simulink model "sm_aileron_actuator_2"  (R2022b)
settings: Solver=FixedStepAuto  StartTime=0.0  StopTime=50.0  FixedStep=0.01  RelTol=1e-3  AbsTol=1e-4  EnableMultiTasking=on
PostLoadFcn:
  | warning('off','sm:sli:setup:compile:LocalSolverNotSupported')
StartFcn:
  | tic
StopFcn:
  | Elapsed_Sim_Time = toc;
model workspace: external: MATLAB File aileronAssembly_DataFile.m (data not in the file)
undefined symbols (not defined in the file or in its folder): AAC_Param, ang2Ext_coeff, Ki, Ki_scaling_elec, Kp, Leadscrew, motor_friction, R7_sctrl, sigbuilder_block, sm_aileron_actuator_lib, smiData, X, Y, Z
libraries: sm_lib x608, fl_lib x380, ee_lib x103, nesl_utility x87, sh_lib x7, sdl_lib x3, simulink x2, slpidlib x2
(part 22 of 22)

== system sm_aileron_actuator_2/Actuator/Electric/Leadscrew 2/Control/Circuit/Current Controller/PS2V ==
  Controlled Voltage Source : fl_lib/Electrical/Electrical Sources/Controlled Voltage Source
  Electrical Reference : fl_lib/Electrical/Electrical Elements/Electrical Reference
  PS : PMIOPort  Side=Right
  V : PMIOPort  Port=2  Side=Left
  connections:
  V/RConn1 -- Controlled Voltage Source/LConn1
  PS/RConn1 -- Controlled Voltage Source/RConn1
  Electrical Reference/LConn1 -- Controlled Voltage Source/RConn2

== system sm_aileron_actuator_2/Actuator/Electric/Leadscrew 2/Control/Simulink/Current Controller/SL2V_1 ==
  SL : Inport
  Controlled Voltage Source : fl_lib/Electrical/Electrical Sources/Controlled Voltage Source
  Electrical Reference : fl_lib/Electrical/Electrical Elements/Electrical Reference
  Simulink-PS Converter : nesl_utility/Simulink-PS Converter  PhysicalDomain=network_engine_domain  SubClassName=ps_input  LeftPortType=input  RightPortType=output  PseudoPeriodic=off  Frequencies=[]  NoiseDistribution=none  NoiseParameters=[]  Unit=V  AffineConversion=off  FilteringAndDerivatives=zero  SimscapeFilterOrder=1  InputFilterTimeConstant=0.005  UdotUserProvided=0
  V : PMIOPort  Side=Right
  wires:
  SL/1 -> Simulink-PS Converter/1
  connections:
  Simulink-PS Converter/RConn1 -- Controlled Voltage Source/RConn1
  V/RConn1 -- Controlled Voltage Source/LConn1
  Electrical Reference/LConn1 -- Controlled Voltage Source/RConn2

== system sm_aileron_actuator_2/Actuator/Electric/Leadscrew 2/Control/Simulink/Current Controller/SL2V_2 ==
  SL : Inport
  Controlled Voltage Source : fl_lib/Electrical/Electrical Sources/Controlled Voltage Source
  Electrical Reference : fl_lib/Electrical/Electrical Elements/Electrical Reference
  Simulink-PS Converter : nesl_utility/Simulink-PS Converter  PhysicalDomain=network_engine_domain  SubClassName=ps_input  LeftPortType=input  RightPortType=output  PseudoPeriodic=off  Frequencies=[]  NoiseDistribution=none  NoiseParameters=[]  Unit=V  AffineConversion=off  FilteringAndDerivatives=zero  SimscapeFilterOrder=1  InputFilterTimeConstant=0.005  UdotUserProvided=0
  V : PMIOPort  Side=Right
  wires:
  SL/1 -> Simulink-PS Converter/1
  connections:
  Electrical Reference/LConn1 -- Controlled Voltage Source/RConn2
  V/RConn1 -- Controlled Voltage Source/LConn1
  Simulink-PS Converter/RConn1 -- Controlled Voltage Source/RConn1

== system sm_aileron_actuator_2/Actuator/Electric/Leadscrew 2/Hall Effect Sensor/Detailed Sensor/PIC Decoder/Pulse decode ==
  A : Inport
  B : Inport  Port=2
  Clock : Clock
  Constant : Constant  Value=0.5
  Sign : Signum
  Sum1 : Sum  Inputs=|-+
  Triggered Subsystem : Subsystem  TreatAsAtomicUnit=on
  Pulse frequency : Outport  VectorParamsAs1DForOutWhenUnconnected=off
  Direction : Outport  Port=2  VectorParamsAs1DForOutWhenUnconnected=off
  Pulse count : Outport  Port=3  VectorParamsAs1DForOutWhenUnconnected=off
  wires:
  Constant/1 -> Sum1/2
  Sum1/1 -> Sign/1
  B/1 -> Sum1/1
  Sign/1 -> Triggered Subsystem/1(sign)
  A/1 -> Triggered Subsystem/Trigger
  Triggered Subsystem/1(Pulse count) -> Pulse count/1
  Clock/1 -> Triggered Subsystem/2(clk)
  Triggered Subsystem/2(Pulse frequency) -> Pulse frequency/1
  Triggered Subsystem/3(Direction) -> Direction/1

== system sm_aileron_actuator_2/Actuator/Electric/Leadscrew 2/Hall Effect Sensor/Detailed Sensor/PIC Decoder/V2SL_1 ==
  Electrical Reference1 : fl_lib/Electrical/Electrical Elements/Electrical Reference
  PS-Simulink Converter 2 : nesl_utility/PS-Simulink Converter  PhysicalDomain=network_engine_domain  SubClassName=ps_output  LeftPortType=input  RightPortType=output  PseudoPeriodic=off  Frequencies=[]  VectorFormat=1-D array  Unit=V  AffineConversion=off
  V2logic : Gain  Gain=0.2
  Voltage Sensor : fl_lib/Electrical/Electrical Sensors/Voltage Sensor
  V : PMIOPort  Side=Left
  SL : Outport  VectorParamsAs1DForOutWhenUnconnected=off
  wires:
  V2logic/1 -> SL/1
  PS-Simulink Converter 2/1 -> V2logic/1
  connections:
  Voltage Sensor/RConn1 -- PS-Simulink Converter 2/LConn1
  V/RConn1 -- Voltage Sensor/LConn1
  Voltage Sensor/RConn2 -- Electrical Reference1/LConn1

== system sm_aileron_actuator_2/Actuator/Electric/Leadscrew 2/Hall Effect Sensor/Detailed Sensor/PIC Decoder/V2SL_2 ==
  Electrical Reference1 : fl_lib/Electrical/Electrical Elements/Electrical Reference
  PS-Simulink Converter 2 : nesl_utility/PS-Simulink Converter  PhysicalDomain=network_engine_domain  SubClassName=ps_output  LeftPortType=input  RightPortType=output  PseudoPeriodic=off  Frequencies=[]  VectorFormat=1-D array  Unit=V  AffineConversion=off
  V2logic : Gain  Gain=0.2
  Voltage Sensor : fl_lib/Electrical/Electrical Sensors/Voltage Sensor
  V : PMIOPort  Side=Left
  SL : Outport  VectorParamsAs1DForOutWhenUnconnected=off
  wires:
  PS-Simulink Converter 2/1 -> V2logic/1
  V2logic/1 -> SL/1
  connections:
  Voltage Sensor/RConn2 -- Electrical Reference1/LConn1
  V/RConn1 -- Voltage Sensor/LConn1
  Voltage Sensor/RConn1 -- PS-Simulink Converter 2/LConn1

== system sm_aileron_actuator_2/Actuator/Electric/Leadscrew 2/Motor Driver/Circuit/LegNl/Sensor Voltage ==
  Goto : Goto  Commented=on  GotoTag=Vds_M2  TagVisibility=global
  PS-Simulink : nesl_utility/PS-Simulink Converter  PhysicalDomain=network_engine_domain  SubClassName=ps_output  LeftPortType=input  RightPortType=output  PseudoPeriodic=off  Frequencies=[]  VectorFormat=1-D array  Unit=V  AffineConversion=off
  Voltage Sensor : fl_lib/Electrical/Electrical Sensors/Voltage Sensor
  + : PMIOPort  Side=Left
  - : PMIOPort  Port=2  Side=Right
  wires:
  PS-Simulink/1 -> Goto/1
  connections:
  -/RConn1 -- Voltage Sensor/RConn2
  +/RConn1 -- Voltage Sensor/LConn1
  Voltage Sensor/RConn1 -- PS-Simulink/LConn1

== system sm_aileron_actuator_2/Actuator/Electric/Leadscrew 2/Motor Driver/Circuit/LegNu/Sensor Voltage ==
  Goto : Goto  Commented=on  GotoTag=Vds_M4  TagVisibility=global
  PS-Simulink : nesl_utility/PS-Simulink Converter  PhysicalDomain=network_engine_domain  SubClassName=ps_output  LeftPortType=input  RightPortType=output  PseudoPeriodic=off  Frequencies=[]  VectorFormat=1-D array  Unit=V  AffineConversion=off
  Voltage Sensor : fl_lib/Electrical/Electrical Sensors/Voltage Sensor
  + : PMIOPort  Side=Left
  - : PMIOPort  Port=2  Side=Right
  wires:
  PS-Simulink/1 -> Goto/1
  connections:
  Voltage Sensor/RConn1 -- PS-Simulink/LConn1
  +/RConn1 -- Voltage Sensor/LConn1
  -/RConn1 -- Voltage Sensor/RConn2

== system sm_aileron_actuator_2/Actuator/Electric/Leadscrew 2/Motor Driver/Circuit/LegPl/Sensor Voltage ==
  Goto : Goto  Commented=on  GotoTag=Vds_M1  TagVisibility=global
  PS-Simulink : nesl_utility/PS-Simulink Converter  PhysicalDomain=network_engine_domain  SubClassName=ps_output  LeftPortType=input  RightPortType=output  PseudoPeriodic=off  Frequencies=[]  VectorFormat=1-D array  Unit=V  AffineConversion=off
  Voltage Sensor : fl_lib/Electrical/Electrical Sensors/Voltage Sensor
  + : PMIOPort  Side=Left
  - : PMIOPort  Port=2  Side=Right
  wires:
  PS-Simulink/1 -> Goto/1
  connections:
  Voltage Sensor/RConn1 -- PS-Simulink/LConn1
  +/RConn1 -- Voltage Sensor/LConn1
  -/RConn1 -- Voltage Sensor/RConn2

== system sm_aileron_actuator_2/Actuator/Electric/Leadscrew 2/Motor Driver/Circuit/LegPu/Sensor Pwr ==
  Goto1 : Goto  Commented=on  GotoTag=Power_M3  TagVisibility=global
  PS-Simulink : nesl_utility/PS-Simulink Converter  PhysicalDomain=network_engine_domain  SubClassName=ps_output  LeftPortType=input  RightPortType=output  PseudoPeriodic=off  Frequencies=[]  VectorFormat=1-D array  Unit=W  AffineConversion=off
  Power Sensor : ee_lib/Sensors & Transducers/Power Sensor  measurement_type=1  averaging_period=1e-4 s
  S : PMIOPort  Side=Right
  + : PMIOPort  Port=2  Side=Left
  - : PMIOPort  Port=3  Side=Left
  wires:
  PS-Simulink/1 -> Goto1/1
  connections:
  PS-Simulink/LConn1 -- Power Sensor/RConn1
  Power Sensor/LConn1 -- S/RConn1
  Power Sensor/LConn3 -- -/RConn1
  Power Sensor/LConn2 -- +/RConn1

== system sm_aileron_actuator_2/Actuator/Electric/Leadscrew 2/Motor Driver/Circuit/LegPu/Sensor Voltage ==
  Goto : Goto  Commented=on  GotoTag=Vds_M3  TagVisibility=global
  PS-Simulink : nesl_utility/PS-Simulink Converter  PhysicalDomain=network_engine_domain  SubClassName=ps_output  LeftPortType=input  RightPortType=output  PseudoPeriodic=off  Frequencies=[]  VectorFormat=1-D array  Unit=V  AffineConversion=off
  Voltage Sensor : fl_lib/Electrical/Electrical Sensors/Voltage Sensor
  + : PMIOPort  Side=Left
  - : PMIOPort  Port=2  Side=Right
  wires:
  PS-Simulink/1 -> Goto/1
  connections:
  -/RConn1 -- Voltage Sensor/RConn2
  +/RConn1 -- Voltage Sensor/LConn1
  Voltage Sensor/RConn1 -- PS-Simulink/LConn1

== system sm_aileron_actuator_2/Actuator/Electric/Leadscrew 3/Control/Circuit/Current Controller/PS2V ==
  Controlled Voltage Source : fl_lib/Electrical/Electrical Sources/Controlled Voltage Source
  Electrical Reference : fl_lib/Electrical/Electrical Elements/Electrical Reference
  PS : PMIOPort  Side=Right
  V : PMIOPort  Port=2  Side=Left
  connections:
  V/RConn1 -- Controlled Voltage Source/LConn1
  PS/RConn1 -- Controlled Voltage Source/RConn1
  Electrical Reference/LConn1 -- Controlled Voltage Source/RConn2

== system sm_aileron_actuator_2/Actuator/Electric/Leadscrew 3/Control/Simulink/Current Controller/SL2V_1 ==
  SL : Inport
  Controlled Voltage Source : fl_lib/Electrical/Electrical Sources/Controlled Voltage Source
  Electrical Reference : fl_lib/Electrical/Electrical Elements/Electrical Reference
  Simulink-PS Converter : nesl_utility/Simulink-PS Converter  PhysicalDomain=network_engine_domain  SubClassName=ps_input  LeftPortType=input  RightPortType=output  PseudoPeriodic=off  Frequencies=[]  NoiseDistribution=none  NoiseParameters=[]  Unit=V  AffineConversion=off  FilteringAndDerivatives=zero  SimscapeFilterOrder=1  InputFilterTimeConstant=0.005  UdotUserProvided=0
  V : PMIOPort  Side=Right
  wires:
  SL/1 -> Simulink-PS Converter/1
  connections:
  Simulink-PS Converter/RConn1 -- Controlled Voltage Source/RConn1
  V/RConn1 -- Controlled Voltage Source/LConn1
  Electrical Reference/LConn1 -- Controlled Voltage Source/RConn2

== system sm_aileron_actuator_2/Actuator/Electric/Leadscrew 3/Control/Simulink/Current Controller/SL2V_2 ==
  SL : Inport
  Controlled Voltage Source : fl_lib/Electrical/Electrical Sources/Controlled Voltage Source
  Electrical Reference : fl_lib/Electrical/Electrical Elements/Electrical Reference
  Simulink-PS Converter : nesl_utility/Simulink-PS Converter  PhysicalDomain=network_engine_domain  SubClassName=ps_input  LeftPortType=input  RightPortType=output  PseudoPeriodic=off  Frequencies=[]  NoiseDistribution=none  NoiseParameters=[]  Unit=V  AffineConversion=off  FilteringAndDerivatives=zero  SimscapeFilterOrder=1  InputFilterTimeConstant=0.005  UdotUserProvided=0
  V : PMIOPort  Side=Right
  wires:
  SL/1 -> Simulink-PS Converter/1
  connections:
  Electrical Reference/LConn1 -- Controlled Voltage Source/RConn2
  V/RConn1 -- Controlled Voltage Source/LConn1
  Simulink-PS Converter/RConn1 -- Controlled Voltage Source/RConn1

== system sm_aileron_actuator_2/Actuator/Electric/Leadscrew 3/Hall Effect Sensor/Detailed Sensor/PIC Decoder/Pulse decode ==
  A : Inport
  B : Inport  Port=2
  Clock : Clock
  Constant : Constant  Value=0.5
  Sign : Signum
  Sum1 : Sum  Inputs=|-+
  Triggered Subsystem : Subsystem  TreatAsAtomicUnit=on
  Pulse frequency : Outport  VectorParamsAs1DForOutWhenUnconnected=off
  Direction : Outport  Port=2  VectorParamsAs1DForOutWhenUnconnected=off
  Pulse count : Outport  Port=3  VectorParamsAs1DForOutWhenUnconnected=off
  wires:
  Constant/1 -> Sum1/2
  Sum1/1 -> Sign/1
  B/1 -> Sum1/1
  Sign/1 -> Triggered Subsystem/1(sign)
  A/1 -> Triggered Subsystem/Trigger
  Triggered Subsystem/1(Pulse count) -> Pulse count/1
  Clock/1 -> Triggered Subsystem/2(clk)
  Triggered Subsystem/2(Pulse frequency) -> Pulse frequency/1
  Triggered Subsystem/3(Direction) -> Direction/1

== system sm_aileron_actuator_2/Actuator/Electric/Leadscrew 3/Hall Effect Sensor/Detailed Sensor/PIC Decoder/V2SL_1 ==
  Electrical Reference1 : fl_lib/Electrical/Electrical Elements/Electrical Reference
  PS-Simulink Converter 2 : nesl_utility/PS-Simulink Converter  PhysicalDomain=network_engine_domain  SubClassName=ps_output  LeftPortType=input  RightPortType=output  PseudoPeriodic=off  Frequencies=[]  VectorFormat=1-D array  Unit=V  AffineConversion=off
  V2logic : Gain  Gain=0.2
  Voltage Sensor : fl_lib/Electrical/Electrical Sensors/Voltage Sensor
  V : PMIOPort  Side=Left
  SL : Outport  VectorParamsAs1DForOutWhenUnconnected=off
  wires:
  V2logic/1 -> SL/1
  PS-Simulink Converter 2/1 -> V2logic/1
  connections:
  Voltage Sensor/RConn1 -- PS-Simulink Converter 2/LConn1
  V/RConn1 -- Voltage Sensor/LConn1
  Voltage Sensor/RConn2 -- Electrical Reference1/LConn1

== system sm_aileron_actuator_2/Actuator/Electric/Leadscrew 3/Hall Effect Sensor/Detailed Sensor/PIC Decoder/V2SL_2 ==
  Electrical Reference1 : fl_lib/Electrical/Electrical Elements/Electrical Reference
  PS-Simulink Converter 2 : nesl_utility/PS-Simulink Converter  PhysicalDomain=network_engine_domain  SubClassName=ps_output  LeftPortType=input  RightPortType=output  PseudoPeriodic=off  Frequencies=[]  VectorFormat=1-D array  Unit=V  AffineConversion=off
  V2logic : Gain  Gain=0.2
  Voltage Sensor : fl_lib/Electrical/Electrical Sensors/Voltage Sensor
  V : PMIOPort  Side=Left
  SL : Outport  VectorParamsAs1DForOutWhenUnconnected=off
  wires:
  PS-Simulink Converter 2/1 -> V2logic/1
  V2logic/1 -> SL/1
  connections:
  Voltage Sensor/RConn2 -- Electrical Reference1/LConn1
  V/RConn1 -- Voltage Sensor/LConn1
  Voltage Sensor/RConn1 -- PS-Simulink Converter 2/LConn1

== system sm_aileron_actuator_2/Actuator/Electric/Leadscrew 3/Motor Driver/Circuit/LegNl/Sensor Voltage ==
  Goto : Goto  Commented=on  GotoTag=Vds_M2  TagVisibility=global
  PS-Simulink : nesl_utility/PS-Simulink Converter  PhysicalDomain=network_engine_domain  SubClassName=ps_output  LeftPortType=input  RightPortType=output  PseudoPeriodic=off  Frequencies=[]  VectorFormat=1-D array  Unit=V  AffineConversion=off
  Voltage Sensor : fl_lib/Electrical/Electrical Sensors/Voltage Sensor
  + : PMIOPort  Side=Left
  - : PMIOPort  Port=2  Side=Right
  wires:
  PS-Simulink/1 -> Goto/1
  connections:
  -/RConn1 -- Voltage Sensor/RConn2
  +/RConn1 -- Voltage Sensor/LConn1
  Voltage Sensor/RConn1 -- PS-Simulink/LConn1

== system sm_aileron_actuator_2/Actuator/Electric/Leadscrew 3/Motor Driver/Circuit/LegNu/Sensor Voltage ==
  Goto : Goto  Commented=on  GotoTag=Vds_M4  TagVisibility=global
  PS-Simulink : nesl_utility/PS-Simulink Converter  PhysicalDomain=network_engine_domain  SubClassName=ps_output  LeftPortType=input  RightPortType=output  PseudoPeriodic=off  Frequencies=[]  VectorFormat=1-D array  Unit=V  AffineConversion=off
  Voltage Sensor : fl_lib/Electrical/Electrical Sensors/Voltage Sensor
  + : PMIOPort  Side=Left
  - : PMIOPort  Port=2  Side=Right
  wires:
  PS-Simulink/1 -> Goto/1
  connections:
  Voltage Sensor/RConn1 -- PS-Simulink/LConn1
  +/RConn1 -- Voltage Sensor/LConn1
  -/RConn1 -- Voltage Sensor/RConn2

== system sm_aileron_actuator_2/Actuator/Electric/Leadscrew 3/Motor Driver/Circuit/LegPl/Sensor Voltage ==
  Goto : Goto  Commented=on  GotoTag=Vds_M1  TagVisibility=global
  PS-Simulink : nesl_utility/PS-Simulink Converter  PhysicalDomain=network_engine_domain  SubClassName=ps_output  LeftPortType=input  RightPortType=output  PseudoPeriodic=off  Frequencies=[]  VectorFormat=1-D array  Unit=V  AffineConversion=off
  Voltage Sensor : fl_lib/Electrical/Electrical Sensors/Voltage Sensor
  + : PMIOPort  Side=Left
  - : PMIOPort  Port=2  Side=Right
  wires:
  PS-Simulink/1 -> Goto/1
  connections:
  Voltage Sensor/RConn1 -- PS-Simulink/LConn1
  +/RConn1 -- Voltage Sensor/LConn1
  -/RConn1 -- Voltage Sensor/RConn2

== system sm_aileron_actuator_2/Actuator/Electric/Leadscrew 3/Motor Driver/Circuit/LegPu/Sensor Pwr ==
  Goto1 : Goto  Commented=on  GotoTag=Power_M3  TagVisibility=global
  PS-Simulink : nesl_utility/PS-Simulink Converter  PhysicalDomain=network_engine_domain  SubClassName=ps_output  LeftPortType=input  RightPortType=output  PseudoPeriodic=off  Frequencies=[]  VectorFormat=1-D array  Unit=W  AffineConversion=off
  Power Sensor : ee_lib/Sensors & Transducers/Power Sensor  measurement_type=1  averaging_period=1e-4 s
  S : PMIOPort  Side=Right
  + : PMIOPort  Port=2  Side=Left
  - : PMIOPort  Port=3  Side=Left
  wires:
  PS-Simulink/1 -> Goto1/1
  connections:
  PS-Simulink/LConn1 -- Power Sensor/RConn1
  Power Sensor/LConn1 -- S/RConn1
  Power Sensor/LConn3 -- -/RConn1
  Power Sensor/LConn2 -- +/RConn1

== system sm_aileron_actuator_2/Actuator/Electric/Leadscrew 3/Motor Driver/Circuit/LegPu/Sensor Voltage ==
  Goto : Goto  Commented=on  GotoTag=Vds_M3  TagVisibility=global
  PS-Simulink : nesl_utility/PS-Simulink Converter  PhysicalDomain=network_engine_domain  SubClassName=ps_output  LeftPortType=input  RightPortType=output  PseudoPeriodic=off  Frequencies=[]  VectorFormat=1-D array  Unit=V  AffineConversion=off
  Voltage Sensor : fl_lib/Electrical/Electrical Sensors/Voltage Sensor
  + : PMIOPort  Side=Left
  - : PMIOPort  Port=2  Side=Right
  wires:
  PS-Simulink/1 -> Goto/1
  connections:
  -/RConn1 -- Voltage Sensor/RConn2
  +/RConn1 -- Voltage Sensor/LConn1
  Voltage Sensor/RConn1 -- PS-Simulink/LConn1

== system sm_aileron_actuator_2/Actuator/Electric/Leadscrew 1/Hall Effect Sensor/Detailed Sensor/PIC Decoder/Pulse decode/Triggered Subsystem ==
  sign : Inport
  clk : Inport  Port=2
  Trigger : TriggerPort  VariantControl=Variant
  Math Function : Math  Operator=reciprocal  SignedPower=on
  Sum : Sum  Inputs=|+-
  Sum1 : Sum  Inputs=|++
  Unit Delay : UnitDelay  SampleTime=-1  HasFrameUpgradeWarning=on
  Unit Delay1 : UnitDelay  InitialCondition=-1e10  SampleTime=-1  HasFrameUpgradeWarning=on
  Pulse count : Outport  InitialOutput=0  VectorParamsAs1DForOutWhenUnconnected=off
  Pulse frequency : Outport  Port=2  VectorParamsAs1DForOutWhenUnconnected=off
  Direction : Outport  Port=3  InitialOutput=0  VectorParamsAs1DForOutWhenUnconnected=off
  wires:
  Sum1/1 -> Unit Delay/1
  sign/1 -> Sum1/1, Direction/1
  Unit Delay/1 -> Pulse count/1, Sum1/2
  clk/1 -> Unit Delay1/1, Sum/1
  Unit Delay1/1 -> Sum/2
  Sum/1 -> Math Function/1
  Math Function/1 -> Pulse frequency/1

== system sm_aileron_actuator_2/Actuator/Electric/Leadscrew 2/Hall Effect Sensor/Detailed Sensor/PIC Decoder/Pulse decode/Triggered Subsystem ==
  sign : Inport
  clk : Inport  Port=2
  Trigger : TriggerPort  VariantControl=Variant
  Math Function : Math  Operator=reciprocal  SignedPower=on
  Sum : Sum  Inputs=|+-
  Sum1 : Sum  Inputs=|++
  Unit Delay : UnitDelay  SampleTime=-1  HasFrameUpgradeWarning=on
  Unit Delay1 : UnitDelay  InitialCondition=-1e10  SampleTime=-1  HasFrameUpgradeWarning=on
  Pulse count : Outport  InitialOutput=0  VectorParamsAs1DForOutWhenUnconnected=off
  Pulse frequency : Outport  Port=2  VectorParamsAs1DForOutWhenUnconnected=off
  Direction : Outport  Port=3  InitialOutput=0  VectorParamsAs1DForOutWhenUnconnected=off
  wires:
  Sum1/1 -> Unit Delay/1
  sign/1 -> Sum1/1, Direction/1
  Unit Delay/1 -> Pulse count/1, Sum1/2
  clk/1 -> Unit Delay1/1, Sum/1
  Unit Delay1/1 -> Sum/2
  Sum/1 -> Math Function/1
  Math Function/1 -> Pulse frequency/1

== system sm_aileron_actuator_2/Actuator/Electric/Leadscrew 3/Hall Effect Sensor/Detailed Sensor/PIC Decoder/Pulse decode/Triggered Subsystem ==
  sign : Inport
  clk : Inport  Port=2
  Trigger : TriggerPort  VariantControl=Variant
  Math Function : Math  Operator=reciprocal  SignedPower=on
  Sum : Sum  Inputs=|+-
  Sum1 : Sum  Inputs=|++
  Unit Delay : UnitDelay  SampleTime=-1  HasFrameUpgradeWarning=on
  Unit Delay1 : UnitDelay  InitialCondition=-1e10  SampleTime=-1  HasFrameUpgradeWarning=on
  Pulse count : Outport  InitialOutput=0  VectorParamsAs1DForOutWhenUnconnected=off
  Pulse frequency : Outport  Port=2  VectorParamsAs1DForOutWhenUnconnected=off
  Direction : Outport  Port=3  InitialOutput=0  VectorParamsAs1DForOutWhenUnconnected=off
  wires:
  Sum1/1 -> Unit Delay/1
  sign/1 -> Sum1/1, Direction/1
  Unit Delay/1 -> Pulse count/1, Sum1/2
  clk/1 -> Unit Delay1/1, Sum/1
  Unit Delay1/1 -> Sum/2
  Sum/1 -> Math Function/1
  Math Function/1 -> Pulse frequency/1

== stateflow chart sm_aileron_actuator_2/Actuator/Electric/Stateflow_2 ==
  state constant_angle
    S = 0;
  state Retract1
  state Extend1
  state Retract2
  state Extend2
  state Retract3
  state Extend3
  state Retract4
  state Extend4
  state Retraction
    S =1;
  state Extension
    S = -1;
  (default) -> constant_angle
  constant_angle -> Retract1 [order 1] : [del_qCmd > 0]
  constant_angle -> Extend1 [order 2] : [del_qCmd < 0]
  Retraction -> constant_angle [order 2] : [del_qCmd == 0]
  Extension -> constant_angle [order 2] : [del_qCmd == 0]
  Retraction -> Extend1 [order 1] : [del_qCmd<0]
  Extension -> Retract1 [order 1] : [del_qCmd>0]
  Retract1 -> Retract2 : [del_I>0]
  Extend1 -> Extend2 : [del_I < 0]
  Retract2 -> Retract3 : [del_fz<0]
  Extend2 -> Extend3 : [del_fz > 0]
  Retract3 -> Retract4 : [del_Disp < 0]
  Extend3 -> Extend4 : [del_Disp > 0]
  Retract4 -> Retraction : [del_qMeas> 0]
  Extend4 -> Extension : [del_qMeas < 0]
  data: del_fz input; del_qMeas input; del_qCmd input; del_Disp input; del_I input; S output

== stateflow chart sm_aileron_actuator_2/Actuator/Electric/Stateflow_3 ==
  state constant_angle
    S = 0;
  state Retract1
  state Extend1
  state Retract2
  state Extend2
  state Retract3
  state Extend3
  state Retract4
  state Extend4
  state Retraction
    S =1;
  state Extension
    S = -1;
  (default) -> constant_angle
  constant_angle -> Retract1 [order 1] : [del_qCmd > 0]
  constant_angle -> Extend1 [order 2] : [del_qCmd < 0]
  Retraction -> constant_angle [order 2] : [del_qCmd == 0]
  Extension -> constant_angle [order 2] : [del_qCmd == 0]
  Retraction -> Extend1 [order 1] : [del_qCmd<0]
  Extension -> Retract1 [order 1] : [del_qCmd>0]
  Retract1 -> Retract2 : [del_I>0]
  Extend1 -> Extend2 : [del_I < 0]
  Retract2 -> Retract3 : [del_fz<0]
  Extend2 -> Extend3 : [del_fz > 0]
  Retract3 -> Retract4 : [del_Disp < 0]
  Extend3 -> Extend4 : [del_Disp > 0]
  Retract4 -> Retraction : [del_qMeas> 0]
  Extend4 -> Extension : [del_qMeas < 0]
  data: del_fz input; del_qMeas input; del_qCmd input; del_Disp input; del_I input; S output

== stateflow chart sm_aileron_actuator_2/Actuator/Electric/Stateflow_1 ==
  state constant_angle
    S = 0;
  state Retract1
  state Extend1
  state Retract2
  state Extend2
  state Retract3
  state Extend3
  state Retract4
  state Extend4
  state Retraction
    S =1;
  state Extension
    S = -1;
  (default) -> constant_angle
  constant_angle -> Retract1 [order 1] : [del_qCmd > 0]
  constant_angle -> Extend1 [order 2] : [del_qCmd < 0]
  Retraction -> constant_angle [order 2] : [del_qCmd == 0]
  Extension -> constant_angle [order 2] : [del_qCmd == 0]
  Retraction -> Extend1 [order 1] : [del_qCmd<0]
  Extension -> Retract1 [order 1] : [del_qCmd>0]
  Retract1 -> Retract2 : [del_I>0]
  Extend1 -> Extend2 : [del_I < 0]
  Retract2 -> Retract3 : [del_fz<0]
  Extend2 -> Extend3 : [del_fz > 0]
  Retract3 -> Retract4 : [del_Disp < 0]
  Extend3 -> Extend4 : [del_Disp > 0]
  Retract4 -> Retraction : [del_qMeas> 0]
  Extend4 -> Extension : [del_qMeas < 0]
  data: del_fz input; del_qMeas input; del_qCmd input; del_Disp input; del_I input; S output
